simulink model "Node_N"  (R2024b)
settings: Solver=ode1  StartTime=0.0  StopTime=10.0  FixedStep=0.5e-3  RelTol=1e-3
settings Model: Creator=wai484  LastModifiedBy=wai484
settings SolverCC: EnableFixedStepZeroCrossing=on
settings DataIOCC: SaveOutput=off  SaveTime=off
settings ModelReferenceCC: ModelReferenceMinAlgLoopOccurrences=on
settings GRTTargetCC: CombineOutputUpdateFcns=off

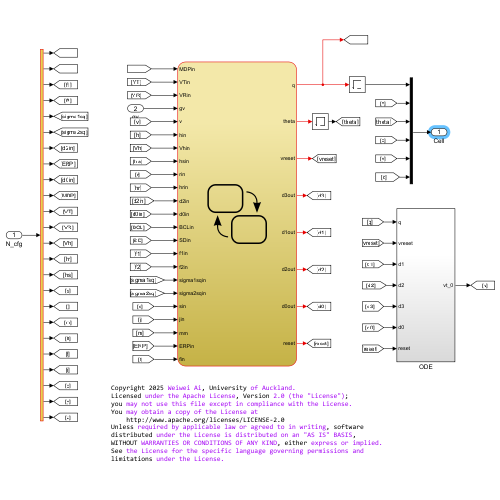
[thumbnail: Simulink's stored preview of the top-level diagram]
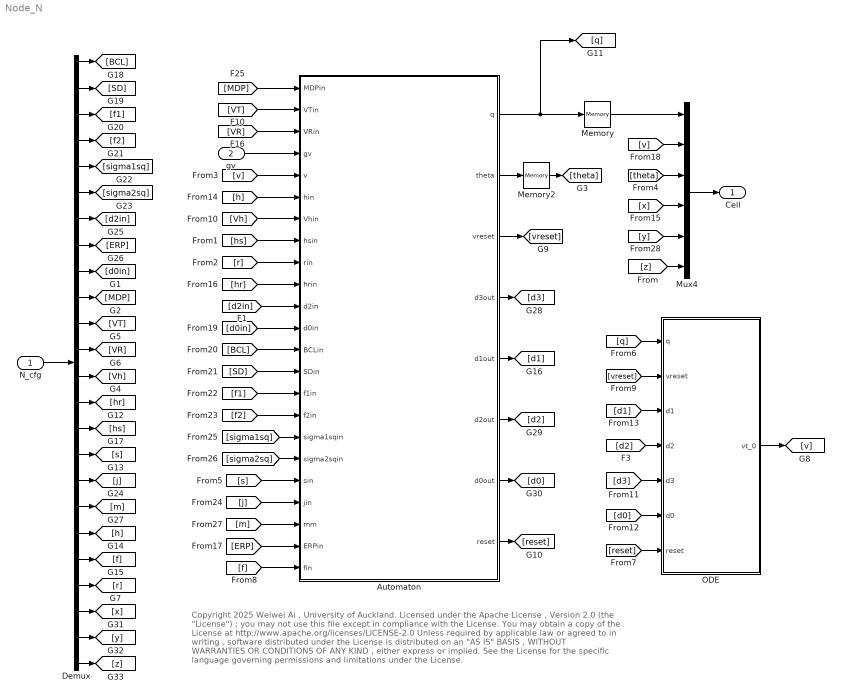
== system Node_N ==
  note: Copyright 2025 Weiwei Ai , University of Auckland.
      | Licensed under the Apache License , Version 2.0 (the "License") ;
      | you may not use this file except in compliance with the License.
      | You may obtain a copy of the License at
      | http://www.apache.org/licenses/LICENSE-2.0
      | Unless required by applicable law or agreed to in writing , software
      | distributed under the License is distributed on an "AS IS" BASIS ,
      | WITHOUT WARRANTIES OR CONDITIONS OF ANY KIND , either express or implied.
      | See the License for the specific language governing permissions and
      | limitations under the License.
  N_cfg : Inport  OutDataTypeStr=double
  gv : Inport  Port=2  OutDataTypeStr=double  PortDimensions=1
  Automaton : Stateflow chart  TreatAsAtomicUnit=on
  Demux : Demux  Outputs=24
  Memory : Memory
  Memory2 : Memory
  Mux4 : Mux  Inputs=6
  ODE : Subsystem
  Cell : Outport  OutDataTypeStr=double
  wires:
  N_cfg/1 -> Demux/1
  Automaton/1(q) -> [q], Memory/1
  Mux4/1 -> Cell/1
  Memory/1 -> Mux4/1
  [VR] -> Automaton/3(VRin)
  [VT] -> Automaton/2(VTin)
  [MDP] -> Automaton/1(MDPin)
  [r] -> Automaton/9(rin)
  [d1] -> ODE/3(d1)
  [d2] -> ODE/4(d2)
  [d3] -> ODE/5(d3)
  [d0] -> ODE/6(d0)
  [v] -> Automaton/5(v)
  ODE/1(vt_0) -> [v]
  Automaton/3(vreset) -> [vreset]
  Automaton/8(reset) -> [reset]
  [q] -> ODE/1(q)
  [reset] -> ODE/7(reset)
  [vreset] -> ODE/2(vreset)
  [Vh] -> Automaton/7(Vhin)
  [hs] -> Automaton/8(hsin)
  [h] -> Automaton/6(hin)
  [hr] -> Automaton/10(hrin)
  [v] -> Mux4/2
  [theta] -> Mux4/3
  Automaton/2(theta) -> Memory2/1
  Memory2/1 -> [theta]
  Automaton/5(d1out) -> [d1]
  [d2in] -> Automaton/11(d2in)
  [d0in] -> Automaton/12(d0in)
  [BCL] -> Automaton/13(BCLin)
  [SD] -> Automaton/14(SDin)
  [f1] -> Automaton/15(f1in)
  [f2] -> Automaton/16(f2in)
  [sigma1sq] -> Automaton/17(sigma1sqin)
  [sigma2sq] -> Automaton/18(sigma2sqin)
  Demux/1 -> [BCL]
  Demux/2 -> [SD]
  Demux/3 -> [f1]
  Demux/4 -> [f2]
  Demux/5 -> [sigma1sq]
  Demux/6 -> [sigma2sq]
  Demux/7 -> [d2in]
  Demux/8 -> [ERP]
  Demux/9 -> [d0in]
  Demux/10 -> [MDP]
  Demux/11 -> [VT]
  Demux/12 -> [VR]
  Demux/16 -> [s]
  Demux/15 -> [hs]
  Demux/14 -> [hr]
  Demux/13 -> [Vh]
  [s] -> Automaton/19(sin)
  [j] -> Automaton/20(jin)
  Demux/17 -> [j]
  Demux/21 -> [r]
  Demux/20 -> [f]
  Demux/19 -> [h]
  Demux/18 -> [m]
  [m] -> Automaton/21(mm)
  [ERP] -> Automaton/22(ERPin)
  Automaton/4(d3out) -> [d3]
  [f] -> Automaton/23(fin)
  Automaton/6(d2out) -> [d2]
  Automaton/7(d0out) -> [d0]
  Demux/22 -> [x]
  Demux/23 -> [y]
  [x] -> Mux4/4
  [y] -> Mux4/5
  gv/1 -> Automaton/4(gv)
  Demux/24 -> [z]
  [z] -> Mux4/6

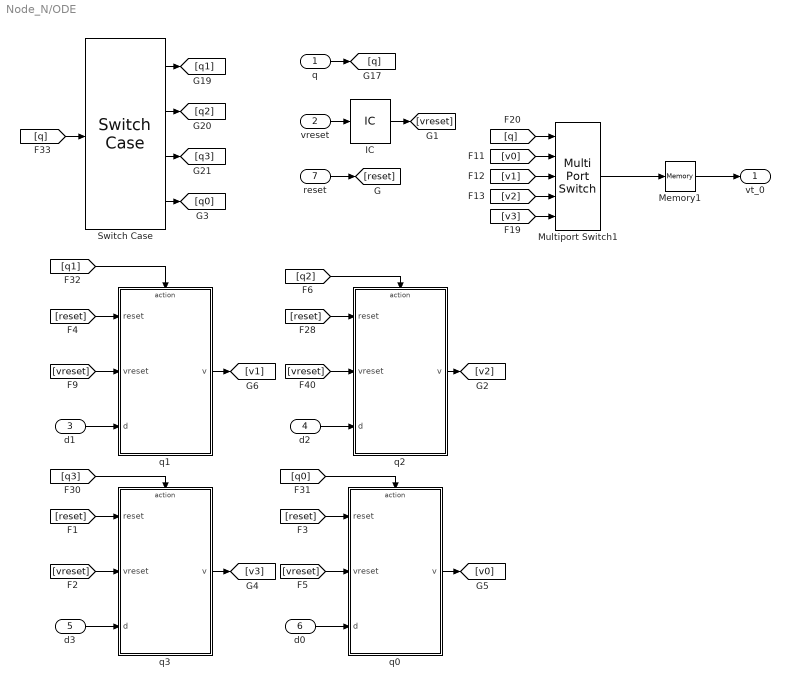
== system Node_N/ODE ==
  q : Inport
  vreset : Inport  Port=2
  d1 : Inport  Port=3
  d2 : Inport  Port=4
  d3 : Inport  Port=5
  d0 : Inport  Port=6
  reset : Inport  Port=7
  IC : InitialCondition  Value=0
  Memory1 : Memory
  Multiport Switch1 : MultiPortSwitch  DataPortOrder=Zero-based contiguous  Inputs=4  zeroidx=on  SaturateOnIntegerOverflow=off  InputSameDT=off
  Switch Case : SwitchCase  CaseConditions={1,2,3,0}  ShowDefaultCase=off
  q0 : Subsystem  TreatAsAtomicUnit=on
  q1 : Subsystem  TreatAsAtomicUnit=on
  q2 : Subsystem  TreatAsAtomicUnit=on
  q3 : Subsystem  TreatAsAtomicUnit=on
  vt_0 : Outport
  wires:
  d1/1 -> q1/3(d)
  [vreset] -> q1/2(vreset)
  [reset] -> q2/1(reset)
  [v3] -> Multiport Switch1/5
  [v2] -> Multiport Switch1/4
  [v1] -> Multiport Switch1/3
  [v0] -> Multiport Switch1/2
  Memory1/1 -> vt_0/1
  [q0] -> q0/Action
  [q3] -> q3/Action
  [vreset] -> q0/2(vreset)
  [reset] -> q0/1(reset)
  d0/1 -> q0/3(d)
  q0/1(v) -> [v0]
  [vreset] -> q3/2(vreset)
  [reset] -> q3/1(reset)
  d3/1 -> q3/3(d)
  q3/1(v) -> [v3]
  [vreset] -> q2/2(vreset)
  [q2] -> q2/Action
  d2/1 -> q2/3(d)
  q2/1(v) -> [v2]
  Switch Case/4 -> [q0]
  Switch Case/3 -> [q3]
  Switch Case/2 -> [q2]
  Switch Case/1 -> [q1]
  [reset] -> q1/1(reset)
  [q1] -> q1/Action
  [q] -> Switch Case/1
  [q] -> Multiport Switch1/1
  q1/1(v) -> [v1]
  q/1 -> [q]
  reset/1 -> [reset]
  vreset/1 -> IC/1
  IC/1 -> [vreset]
  Multiport Switch1/1 -> Memory1/1

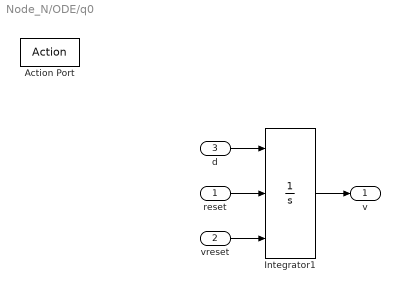
== system Node_N/ODE/q0 ==
  reset : Inport
  vreset : Inport  Port=2
  d : Inport  Port=3
  Action Port : ActionPort  InitializeStates=reset  ActionPortLabel=case [ 0 ]:
  Integrator1 : Integrator  ExternalReset=either  InitialConditionSource=external  InitialCondition=20
  v : Outport
  wires:
  Integrator1/1 -> v/1
  reset/1 -> Integrator1/2
  vreset/1 -> Integrator1/3
  d/1 -> Integrator1/1

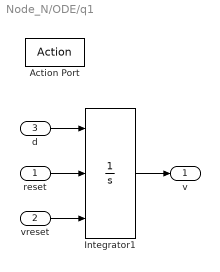
== system Node_N/ODE/q1 ==
  reset : Inport
  vreset : Inport  Port=2
  d : Inport  Port=3
  Action Port : ActionPort  InitializeStates=reset  ActionPortLabel=case [ 1 ]:
  Integrator1 : Integrator  ExternalReset=either  InitialConditionSource=external  InitialCondition=20
  v : Outport
  wires:
  d/1 -> Integrator1/1
  Integrator1/1 -> v/1
  reset/1 -> Integrator1/2
  vreset/1 -> Integrator1/3

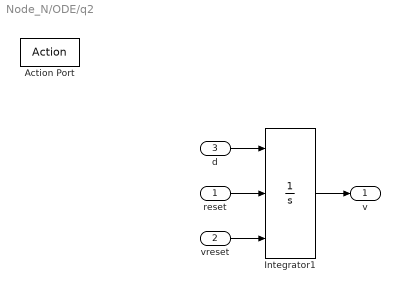
== system Node_N/ODE/q2 ==
  reset : Inport
  vreset : Inport  Port=2
  d : Inport  Port=3
  Action Port : ActionPort  InitializeStates=reset  ActionPortLabel=case [ 2 ]:
  Integrator1 : Integrator  ExternalReset=either  InitialConditionSource=external  InitialCondition=20
  v : Outport
  wires:
  d/1 -> Integrator1/1
  vreset/1 -> Integrator1/3
  reset/1 -> Integrator1/2
  Integrator1/1 -> v/1

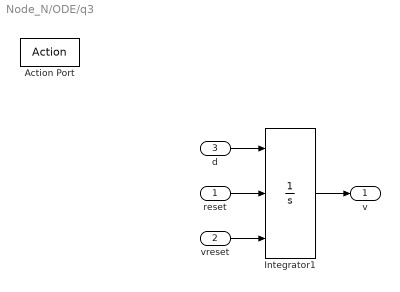
== system Node_N/ODE/q3 ==
  reset : Inport
  vreset : Inport  Port=2
  d : Inport  Port=3
  Action Port : ActionPort  InitializeStates=reset  ActionPortLabel=case [ 3 ]:
  Integrator1 : Integrator  ExternalReset=either  InitialConditionSource=external  InitialCondition=20
  v : Outport
  wires:
  Integrator1/1 -> v/1
  reset/1 -> Integrator1/2
  vreset/1 -> Integrator1/3
  d/1 -> Integrator1/1

== stateflow chart Node_N/Automaton ==
  settings: updateMethod=DISCRETE  executeAtInitialization=1
  state PacemakerCell
    state Cell [parallel]
      settings: executionOrder=1
      state Slow
        en: q=1; %phase4
      state Stimulated
        en: q=2; %phase0
        f1theta=exp(-h*theta);
        Vmax=(-1)*MDP*f1theta;
        [f3theta,n,Vmin]=sat(n,hr,hs,Vh1,s,m,theta);
      state Plateau
        en: q=3;%phase2
      state RP
        en:q=0;%phase3
      (default) -> Slow : /{Vmin=0;Vmax=(-1)*MDP; d3=d3fcn(MDP,VR,VT,d0,d2,ERP); BCL=RR(BCLin,SDin,f1in,f2in,sigma1sqin,sigma2sqin,t);...
          | t3=(abs(MDP)-VR)/abs(d3); t0=VR/abs(d0);t2=(abs(MDP)-VT)/abs(d2);d1=(VT)/(BCL-t3-t0-t2);d1out=d1;}
      Slow -> Stimulated [order 1] : [gv>VT&& v<VT]{theta=(v-VT)/(Vmin-VT);f2theta=exp(-f*theta);d2out=d2*f2theta;...
          |  f4theta=exp(j*(theta-1)); Vh1=Vh*f4theta; n=n+1;  ...
          |  vreset=v;reset; }
      Slow -> Stimulated [order 2] : [v>=VT]{theta=0; f2theta=exp(-f*theta); d2out=d2*f2theta;...
          |  n=(1-r)*n;  vreset=v;reset; }
      RP -> Slow : [v<=Vmin]{t3=(abs(MDP)-VR)/abs(d3); t0=VR/abs(d0);...
          | MDP=MDPin; VT=VTin; d2=d2in; t2=(abs(MDP)-VT)/abs(d2);...
          | BCL=RR(BCLin,SDin,f1in,f2in,sigma1sqin,sigma2sqin,t);...
          | d1=(VT)/(BCL-t3-t0-t2); d1out=d1*f3theta;...
          | VR=VRin; h=hin; Vh=Vhin; hs=hsin; r=rin;hr=hrin;d0=d0in;...
          | s=sin; j=jin; m=mm; ERP=ERPin;f=fin;...
          | vreset=v;reset;}
      Stimulated -> Plateau : [v>=Vmax]{d3=d3fcn(MDP,VR,VT,d0,d2,ERP);...
          | d3out=d3*f2theta;...
          | vreset=v;reset;}
      Plateau -> RP : [v<=VR]{d0out=d0*f2theta; vreset=v;reset;}
    state R [parallel]
      du:
      t=temporalCount(sec);
      settings: executionOrder=2
  (default) -> PacemakerCell : {t=0; MDP=MDPin;VT=VTin;VR=VRin;h=hin;Vh=Vhin;hs=hsin;r=rin;hr=hrin;d2=d2in;d0=d0in;...
      | s=sin;j=jin;m=mm;ERP=ERPin;f=fin;}
  data: f3out function_output double; tout function_output double; pt function_input double; Vminout function_output double; phr function_input double; phs function_input double; pVh function_input double; ps function_input double; pm function_input double; ptheta function_input double; pbcl function_input double; psd function_input double; pf1 function_input double; pf2 function_input double; psigma1sq function_input double; psigma2sq function_input double; rr function_output double size=1; pt function_input double; pMDP function_input double; pVR function_input double; pVT function_input double; pd0 function_input double; pd2 function_input double; pERP function_input double; d3in function_output double; q output double; MDPin input double =0; VTin input double; VRin input; Vmax local double; theta output double; vreset output double; gv input; v input double; hin input double; f1theta local double; Vhin input double; Vh1 local double; hsin input double; rin input double; hrin input double; Vmin local double; d2in input double; d3out output double; d0in input double; BCLin input double; SDin input double; f1in input double; f2in input double; sigma1sqin input double; sigma2sqin input double; d1out output double; Vtemp local double; t local double; sin input double; jin input double; mm input double; ERPin input double; f3theta local double; d2out output double; fin input double; d0out output double; f2theta local double; n local double; f4theta local double; d2 local double; Vh local double; h local double; hr local double; hs local double; j local double; m local double; r local double; s local double; BCL local double; ERP local double; MDP local double; VR local double; VT local double; d0 local double; f local double; d1 local double; d3 local double; t0 local double; t2 local double; t3 local double
  data v settings: updateMethod=SF_CONTINUOUS_TIME_DATA
  events: reset output EITHER_EDGE_EVENT
  function [f3out,tout,Vminout]=sat(pt,phr,phs,pVh,ps,pm,ptheta):
    | function [f3out,tout,Vminout]=sat(pt,phr,phs,pVh,ps,pm,ptheta)
    | 
    | td=phr*(pt-phs);
    | 
    | if td>=5
    |     tout=5/phr+phs;
    | else
    |     tout=pt;
    | end
    | 
    | if tout<1
    | co=0;
    | else
    | Vtemp=1+exp(-phr*(tout-phs)); 
    | co=1/Vtemp;
    | end;
    | Vminout=pVh*co;
    | thetai=ptheta;
    | for i=1:ps-1
    |     thetai=thetai*ptheta;
    | end
    | ft=pm*co*thetai+1;
    | f3out=1/ft;
    | end
  function rr= RR(pbcl,psd,pf1,pf2,psigma1sq,psigma2sq,pt):
    | function rr= RR(pbcl,psd,pf1,pf2,psigma1sq,psigma2sq,pt)
    | %Rate dependent factor
    | c1=0.01;
    | c2=0.01;
    | if psigma1sq<0 || psigma2sq<0
    |     error('Invalid input');
    | end
    | % The Gaussian frequency distribution, power spectrum
    | hf=0.5;
    | fstep=0.025;
    | ff=0:fstep:hf; % The frequency range original;
    | % fmax=1; % Assume the highest frequency
    | % fmin=0.025; % Assume the lowest frequency
    | % Fs=2*fmax; % The sample frequency 
    | % tstep=1/Fs; % The sample period of the time series
    | % tmax=1/fmin; % The period of the time series
    | % N=tmax/tstep;
    | % fstep=2*fmax/N; % =fmin
    | % f=fstep:fstep:fmax; % The frequency range original; 
    | ln=length(ff); % The number of frequency/cos signals.
    | s1=(psigma1sq/(c1*sqrt(2*pi)))*exp(-(ff-pf1).^2/(2*c1^2));
    | s2=(psigma2sq/(c2*sqrt(2*pi)))*exp(-(ff-pf2).^2/(2*c2^2));
    | ss=s1+s2; % s(f)
    | rss=sqrt(ss); %
    | %Construct the time series y(t) from s(f);
    | mag=rss; % the amplitudes;
    | y = ff'*2*pi*pt;
    | y = cos(y);
    | for i=1:ln
    |     y(i,:)=y(i,:)*mag(i);
    | end
    | if ln>1
    |     y1=sum(y);
    | else
    |     y1=y;
    | end
    | rr=pbcl+y1*psd;
    | end
  function d3in= d3fcn(pMDP,pVR,pVT,pd0,pd2,pERP):
    | function d3in= d3fcn(pMDP,pVR,pVT,pd0,pd2,pERP)
    | %#codegen
    | d3in=-(abs(pMDP)-pVR)/(pERP-(abs(pMDP)-pVT)/pd2-pVR/abs(pd0));
